simulink library "THB_P_adapter"  (R2016b)
settings: Solver=ode45  StartTime=0.0  StopTime=10.0  RelTol=1e-3  EnableMultiTasking=on
libraries: carnot x1
settings Model: Creator=lena.frank  LastModifiedBy=drhf
settings DataIOCC: LimitDataPoints=on  SaveFormat=Array  SignalLoggingSaveFormat=ModelDataLogs
settings OptimizationCC: ExpressionDepthLimit=2147483647  LifeSpan=inf
settings DebuggingCC: UnderspecifiedInitializationDetection=Classic  MergeDetectMultiDrivingBlocksExec=none  SolverPrmCheckMsg=warning  FcnCallInpInsideContextMsg=warning  StateNameClashWarn=warning  SFUnexpectedBacktrackingDiag=warning  SFNoUnconditionalDefaultTransitionDiag=warning  SFExecutionAtInitializationDiag=none
settings HardwareCC: ProdBitPerPointer=32  ProdBitPerSizeT=32  ProdBitPerPtrDiffT=32  ProdLargestAtomicFloat=None  ProdIntDivRoundTo=Undefined  ProdEndianess=Unspecified  ProdWordSize=32  ProdHWDeviceType=32-bit Generic
settings ModelReferenceCC: PropagateSignalLabelsOutOfModel=off
settings GRTTargetCC: TargetLangStandard=C89/C90 (ANSI)  GeneratePreprocessorConditionals=Disable all  CombineOutputUpdateFcns=off  GRTInterface=on
settings ConfigComp: CovMetricSettings=dw  CovHtmlReporting=on  CovSaveCumulativeToWorkspaceVar=on  CovSaveSingleToWorkspaceVar=on  CovExternalEMLEnable=off

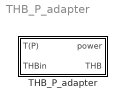
== system THB_P_adapter ==
  THB_P_adapter : Subsystem  mask(ACTIVE COMPONENT){mass=1, ua=800*5*5/0.2*0.022*3.1415, t0=20}
      mask prompts: mass "MASS of fluid in heating element >0, kg"; ua "HEAT TRANSFER of fluid <-> wall >0, W/K"; t0 "start temperature in °C"
      mask help:
      | Adapter between active components and house-model.
      | Transformation from heat flow - defined by the thermo-hydraulic vector THB - to a power entering the block "active wall", "active ceiling", "active floor" or "flat radiator".
      | P  : "electric" power flowing into active layer of wall, W
      | T(P)  : temperature of active layer, °C
      | THB_in  : hydraulic vector input
      | THB_out : hydraulic vector output
      mask init:
      | % mass = str2num(mass);
      | % if length(mass)~=1 error(['PARAMETERS block "' path2block '" : "MASS ..." must have only 1 entry !']); end;
      | % if (mass<=0) error(['PARAMETERS block "' path2block '" : "MASS ..." must be >0 !']); end;
      | % 
      | % ua = str2num(ua);
      | % if length(ua)~=1 error(['PARAMETERS block "' path2block '" : "HEAT TRANSFER ..." must have only 1 entry !']); end;
      | % if (ua<=0) error(['PARAMETERS block "' path2block '" : "HEAT TRANSFER ..." must be >0 !']); end;
      mask Help: web(fullfile(path_carnot('help'),'THB_P_adapter.html'),'-helpbrowser')

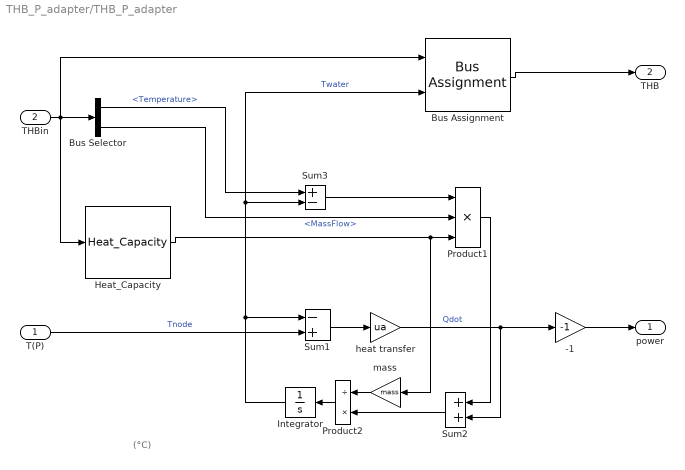
== system THB_P_adapter/THB_P_adapter ==
  note: (°C)
  T(P) : Inport
  THBin : Inport  Port=2
  -1 : Gain  Gain=-1  SaturateOnIntegerOverflow=on  OutDataTypeStr=Inherit: Same as input  ParamDataTypeStr=Inherit: Same as input
  Bus Assignment : BusAssignment  AssignedSignals=Temperature
  Bus Selector : BusSelector  OutputSignals=Temperature,MassFlow
  Heat_Capacity : carnot/Basic/Material_Properties/Heat_Capacity  VariantControl=CarlibClassic  INPUTARGUMENTS=THB  DEBUGLEVEL=DEBUGLEVEL  MAXTOTALWARNINGS=inf  MAXCONSECUTIVEWARNINGS=inf  WRITETOFILE=0  FILENAME='errors.txt'
  Integrator : Integrator  InitialCondition=t0
  Product1 : Product  Inputs=3  SaturateOnIntegerOverflow=on  InputSameDT=on  OutDataTypeStr=Inherit: Same as first input
  Product2 : Product  Inputs=/*  SaturateOnIntegerOverflow=on  InputSameDT=on  OutDataTypeStr=Inherit: Same as first input
  Sum1 : Sum  Inputs=-+  SaturateOnIntegerOverflow=on  InputSameDT=on  OutDataTypeStr=Inherit: Same as first input
  Sum2 : Sum  SaturateOnIntegerOverflow=on  InputSameDT=on  OutDataTypeStr=Inherit: Same as first input
  Sum3 : Sum  Inputs=+-  SaturateOnIntegerOverflow=on  InputSameDT=on  OutDataTypeStr=Inherit: Same as first input
  heat transfer : Gain  Gain=ua  SaturateOnIntegerOverflow=on  OutDataTypeStr=Inherit: Same as input  ParamDataTypeStr=Inherit: Same as input
  mass : Gain  Gain=mass  SaturateOnIntegerOverflow=on  OutDataTypeStr=Inherit: Same as input  ParamDataTypeStr=Inherit: Same as input
  power : Outport
  THB : Outport  Port=2
  wires:
  THBin/1 -> Bus Selector/1, Bus Assignment/1, Heat_Capacity/1
  heat transfer/1 -> -1/1, Sum2/2  "Qdot"
  -1/1 -> power/1
  Sum2/1 -> Product2/2
  Product2/1 -> Integrator/1
  mass/1 -> Product2/1
  Integrator/1 -> Sum3/2, Bus Assignment/2, Sum1/1  "Twater"
  T(P)/1 -> Sum1/2  "Tnode"
  Sum1/1 -> heat transfer/1
  Bus Selector/1 -> Sum3/1  "<Temperature>"
  Heat_Capacity/1 -> mass/1, Product1/3
  Product1/1 -> Sum2/1
  Bus Selector/2 -> Product1/2  "<MassFlow>"
  Sum3/1 -> Product1/1
  Bus Assignment/1 -> THB/1
